simulink model "sns_bridge_reflex"  (R2025b)
settings: Solver=ode45  StartTime=0.0  StopTime=1.5  RelTol=1e-5  AbsTol=1e-7
libraries: SNS_Library x9, mjLib x1
settings Model: Creator=Ben  LastModifiedBy=Ben
settings DataIOCC: SignalLoggingName=sigs

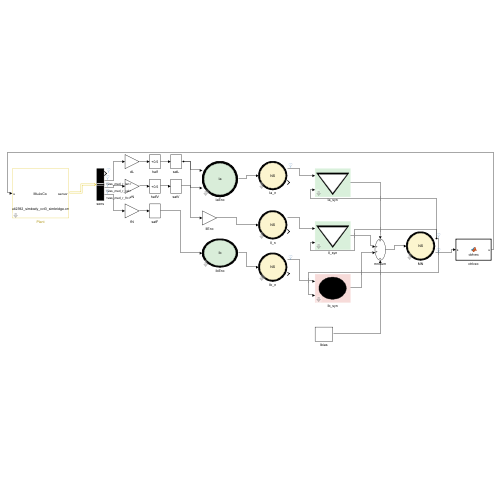
[thumbnail: Simulink's stored preview of the top-level diagram]
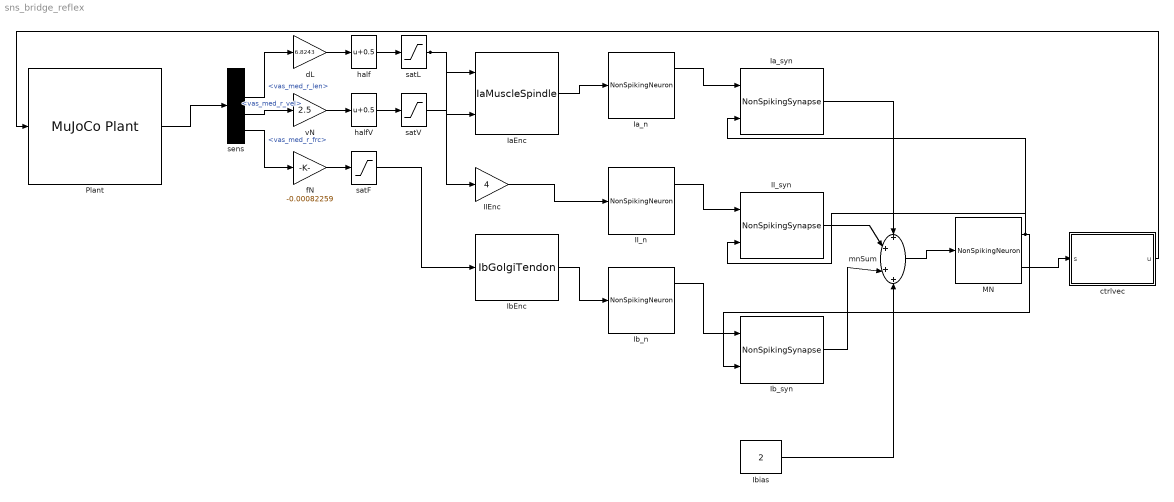
== system sns_bridge_reflex ==
  IIEnc : Gain  Gain=4
  II_n : SNS_Library/NonSpikingNeuron  Vrest=0  Gm=1  Cm=20  Thr=0  Slope=5
  II_syn : SNS_Library/NonSpikingSynapse  gmax=0.4  Esyn=8  ThrPre=0  SlopePre=5
  IaEnc : SNS_Library/IaMuscleSpindle  Imax=10  Wl=4  Wv=8
  Ia_n : SNS_Library/NonSpikingNeuron  Vrest=0  Gm=1  Cm=20  Thr=0  Slope=5
  Ia_syn : SNS_Library/NonSpikingSynapse  gmax=0.6  Esyn=8  ThrPre=0  SlopePre=5
  IbEnc : SNS_Library/IbGolgiTendon  Imax=10  Kf=10
  Ib_n : SNS_Library/NonSpikingNeuron  Vrest=0  Gm=1  Cm=40  Thr=0  Slope=5
  Ib_syn : SNS_Library/NonSpikingSynapse  gmax=0.35  Esyn=-5  ThrPre=0  SlopePre=5
  Ibias : Constant  Value=2
  MN : SNS_Library/NonSpikingNeuron  Vrest=0  Gm=1  Cm=30  Thr=0  Slope=5
  Plant : mjLib/MuJoCo Plant  controlBus=[]  sensorBus=mj_bus_sensor_7979902499018342666  controlLength=[]  sensorLength=[]  rgbLength=[]  depthLength=[]  sampleTime=0.005  xmlFileRel=C:/Users/Ben/Documents/GitHub/Bipedal_Robot/Code/Matlab/SNS_Simscape/mujoco_bridge/matlab/../../../../../Solid_Models/OpenSim/Gait2392_Robotbody/mjc/gait2392_simbody/gait2392_simbody_cvt3_simbridge.xml  xmlFile=C:/Users/Ben/Documents/GitHub/Bipedal_Robot/Code/Matlab/SNS_Simscape/mujoco_bridge/matlab/../../../../../Solid_Models/OpenSim/Gait2392_Robotbody/mjc/gait2392_simbody/gait2392_simbody_cvt3_simbridge.xml  renderingType=None  vsync=off  visualFPS=60  zoomLevel=1  znear=0.02  zfar=100  cameraSampleTime=0.020  rgbOutOption=off  depthOutOption=off  controlInterfaceType=Vector
      settings: SourceProductName=MuJoCo Simulator
  ctrlvec : MATLAB Function  TreatAsAtomicUnit=on
  dL : Gain  Gain=6.8243
  fN : Gain  Gain=-0.00082259
  half : Bias  Bias=0.5  SaturateOnIntegerOverflow=off
  halfV : Bias  Bias=0.5  SaturateOnIntegerOverflow=off
  mnSum : Sum  Inputs=++++
  satF : Saturate  UpperLimit=1  LowerLimit=0
  satL : Saturate  UpperLimit=1  LowerLimit=0
  satV : Saturate  UpperLimit=1  LowerLimit=0
  sens : BusSelector  OutputSignals=knee_r_pos,vas_med_r_len,vas_med_r_vel,vas_med_r_frc
  vN : Gain  Gain=2.5
  wires:
  Plant/1 -> sens/1
  sens/2 -> dL/1  "<vas_med_r_len>"
  dL/1 -> half/1
  half/1 -> satL/1
  sens/3 -> vN/1  "<vas_med_r_vel>"
  vN/1 -> halfV/1
  halfV/1 -> satV/1
  sens/4 -> fN/1  "<vas_med_r_frc>"
  fN/1 -> satF/1
  satL/1 -> IaEnc/1, IIEnc/1
  satV/1 -> IaEnc/2
  satF/1 -> IbEnc/1
  IaEnc/1 -> Ia_n/1
  IIEnc/1 -> II_n/1
  IbEnc/1 -> Ib_n/1
  Ia_n/1 -> Ia_syn/1
  II_n/1 -> II_syn/1
  Ib_n/1 -> Ib_syn/1
  Ia_syn/1 -> mnSum/1
  II_syn/1 -> mnSum/2
  Ib_syn/1 -> mnSum/3
  Ibias/1 -> mnSum/4
  mnSum/1 -> MN/1
  MN/1 -> Ia_syn/2, II_syn/2, Ib_syn/2
  MN/2 -> ctrlvec/1(s)
  ctrlvec/1(u) -> Plant/1

== matlab function sns_bridge_reflex/ctrlvec ==
  data: s input; u output
function u = ctrlvec(s)
%#codegen
u = zeros(92,1); u(29) = s;
